simulink model "room"  (R2024b)
settings: Solver=VariableStepAuto  StartTime=0.0  StopTime=172800  RelTol=1e-3
libraries: fl_lib x9, nesl_utility x5, simulink x2
settings Model: Creator=bhalg  LastModifiedBy=bhalg

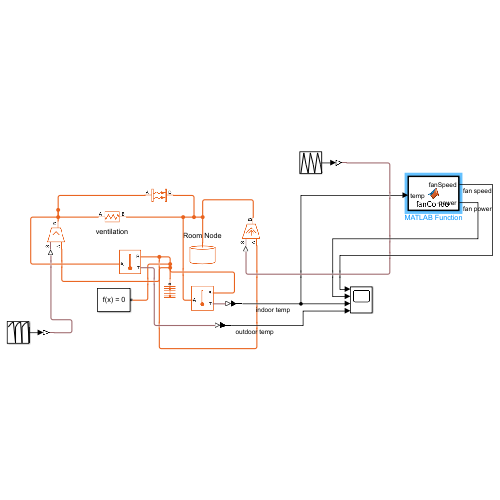
[thumbnail: Simulink's stored preview of the top-level diagram]
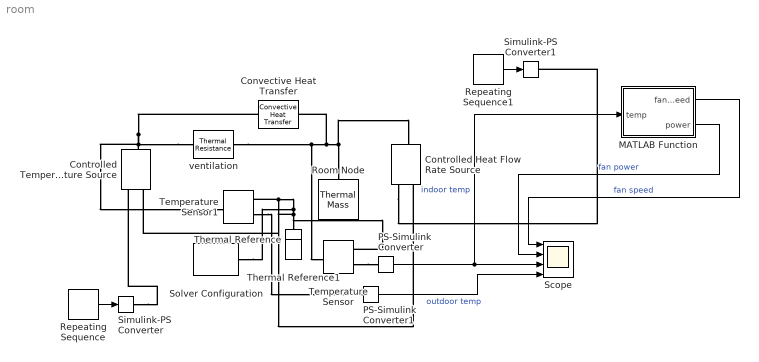
== system room ==
  Controlled Temperature Source : fl_lib/Thermal/Thermal Sources/Controlled Temperature Source
  Controlled Heat Flow Rate Source : fl_lib/Thermal/Thermal Sources/Controlled Heat Flow Rate Source
  Convective Heat Transfer : fl_lib/Thermal/Thermal Elements/Convective Heat Transfer  thermal_type=foundation.enum.constant_variable.constant  area=1 m^2  heat_tr_coeff=2 W/(K*m^2)  min_heat_tr_coeff=1e-3 W/(K*m^2)  T_specify=off  T_priority=None  T=0 K  T_nominal_specify=off  T_nominal_value=1  T_nominal_unit=K  Q_specify=off  Q_priority=None  Q=0 W  Q_nominal_specify=off  Q_nominal_value=1  Q_nominal_unit=W
  MATLAB Function : MATLAB Function  TreatAsAtomicUnit=on
  PS-Simulink Converter : nesl_utility/PS-Simulink Converter  PhysicalDomain=network_engine_domain  SubClassName=ps_output  LeftPortType=input  RightPortType=output  PseudoPeriodic=off  Frequencies=[]  VectorFormat=inherit  Unit=inherit  AffineConversion=off
  PS-Simulink Converter1 : nesl_utility/PS-Simulink Converter  PhysicalDomain=network_engine_domain  SubClassName=ps_output  LeftPortType=input  RightPortType=output  PseudoPeriodic=off  Frequencies=[]  VectorFormat=inherit  Unit=inherit  AffineConversion=off
  Repeating Sequence : simulink/Sources/Repeating Sequence  rep_seq_t=[0 32400 64800 84000]  rep_seq_y=[293 308.15 315.15 227]
  Repeating Sequence1 : simulink/Sources/Repeating Sequence  rep_seq_t=[0 32400 64800 84000]  rep_seq_y=[0 500 200 0]
  Room Node : fl_lib/Thermal/Thermal Elements/Thermal Mass  mass_type=foundation.enum.constant_variable.constant  mass=60 kg  sp_heat=1000 J/(K*kg)  mass_min=1e-6 kg  num_ports=foundation.enum.numPorts2.one  m_specify=off  m_priority=High  m=1 kg  m_nominal_specify=off  m_nominal_value=1  m_nominal_unit=kg  T_specify=on  T_priority=High  T=22 degC  T_nominal_specify=on  T_nominal_value=295.15  T_nominal_unit=K  Q_specify=off  Q_priority=High  Q=0 W  Q_nominal_specify=off  Q_nominal_value=0.1  Q_nominal_unit=W
  Scope : Scope  NumInputPorts=4
  Simulink-PS Converter : nesl_utility/Simulink-PS Converter  PhysicalDomain=network_engine_domain  SubClassName=ps_input  LeftPortType=input  RightPortType=output  PseudoPeriodic=off  Frequencies=[]  NoiseDistribution=none  NoiseParameters=[]  Unit=1  AffineConversion=off  FilteringAndDerivatives=provide  SimscapeFilterOrder=1  InputFilterTimeConstant=0.001  UdotUserProvided=0
  Simulink-PS Converter1 : nesl_utility/Simulink-PS Converter  PhysicalDomain=network_engine_domain  SubClassName=ps_input  LeftPortType=input  RightPortType=output  PseudoPeriodic=off  Frequencies=[]  NoiseDistribution=none  NoiseParameters=[]  Unit=1  AffineConversion=off  FilteringAndDerivatives=provide  SimscapeFilterOrder=1  InputFilterTimeConstant=0.001  UdotUserProvided=0
  Solver Configuration : nesl_utility/Solver Configuration  PhysicalDomain=network_engine_domain  SubClassName=solver  LeftPortType=input  RightPortType=generic  Tones=[]  Harmonics=[]  SimulateNoise=off  Profile=off  UseLocalSampling=off  EnableSwitchedLinearOptims=on  FrequencyDomain=off  UseCCode=off  RelTol=0.001  AbsTol=0.001  MinStep=1e-09  ToWorkspace=off  RevertToSquareIcSolve=off  NumHomotopyIterations=100  PhasorMode=off  PhasorModeNumHarmonics=1  ConsistencySolver=NEWTON_XTOL_AFTER_FTOL  IndexReductionMethod=DerivativeReplacement  DoDC=off  ResidualTolerance=1e-09  ConsistencyTolSource=GLOBAL  ConsistencyAbsTol=0.001  ConsistencyRelTol=0.001  ConsistencyTolFactor=0.001  UseLocalSolver=off  LocalSolverChoice=NE_BACKWARD_EULER_ADVANCER  ResolveIndetEquations=on  FunctionEvalNumThread=1  LocalSolverSampleTime=0.001  DoFixedCost=off  MaxNonlinIter=3  MaxModeIter=2  ComputeImpulses=off  ImpulseIterations=2  LinearAlgebra=auto  LinearAlgebraNumThread=0  EquationFormulation=NE_TIME_EF  DelaysMemoryBudget=1024  AutomaticFiltering=on  FilteringTimeConstant=0.001  PartitionStorageMethod=AS_NEEDED  PartitionMemoryBudget=1024  PartitionMethod=ROBUST  MultibodyUseLocalSolver=off  MultibodyLocalSolverChoice=ODE1  MultibodyLocalSolverSampleTime=0.001
  Temperature Sensor : fl_lib/Thermal/Thermal Sensors/Temperature Sensor  temperature_measure=foundation.enum.MeasurementReference.difference
  Temperature Sensor1 : fl_lib/Thermal/Thermal Sensors/Temperature Sensor  temperature_measure=foundation.enum.MeasurementReference.difference
  Thermal Reference : fl_lib/Thermal/Thermal Elements/Thermal Reference
  Thermal Reference1 : fl_lib/Thermal/Thermal Elements/Thermal Reference
  ventilation : fl_lib/Thermal/Thermal Elements/Thermal Resistance  resistance=2 K/W  T_specify=on  T_priority=High  T=13 degC  T_nominal_specify=on  T_nominal_value=284.15  T_nominal_unit=K  Q_specify=off  Q_priority=High  Q=0 W  Q_nominal_specify=off  Q_nominal_value=0.1  Q_nominal_unit=W
  wires:
  PS-Simulink Converter/1 -> Scope/3, MATLAB Function/1(temp)  "indoor temp"
  PS-Simulink Converter1/1 -> Scope/4  "outdoor temp"
  Repeating Sequence/1 -> Simulink-PS Converter/1
  Repeating Sequence1/1 -> Simulink-PS Converter1/1
  MATLAB Function/2(power) -> Scope/2  "fan power"
  MATLAB Function/1(fanSpeed) -> Scope/1  "fan speed"
  connections:
  ventilation/RConn1 -- Temperature Sensor/LConn1 -- Convective Heat Transfer/RConn1 -- Controlled Heat Flow Rate Source/LConn1 -- Room Node/LConn1
  Temperature Sensor1/RConn1 -- Thermal Reference/LConn1 -- Controlled Temperature Source/RConn2 -- Temperature Sensor/RConn1 -- Solver Configuration/RConn1 -- Controlled Heat Flow Rate Source/RConn2
  Temperature Sensor/RConn2 -- PS-Simulink Converter/LConn1
  ventilation/LConn1 -- Convective Heat Transfer/LConn1 -- Controlled Temperature Source/LConn1 -- Temperature Sensor1/LConn1
  Temperature Sensor1/RConn2 -- PS-Simulink Converter1/LConn1
  Simulink-PS Converter/RConn1 -- Controlled Temperature Source/RConn1
  Controlled Heat Flow Rate Source/RConn1 -- Simulink-PS Converter1/RConn1

== matlab function room/MATLAB Function ==
  data: temp input; fanSpeed output; power output
function [fanSpeed, power] = fanControl(temp)
% fanControl calculates fan speed and power consumption based on temperature
% Inputs:
%   temp - room temperature in °C
% Outputs:
%   fanSpeed - computed fan speed (normalized units)
%   power    - computed power consumption in Watts

% Define parameters
T_ref = 22;       % Reference temperature in °C
S0 = 30;          % Baseline fan speed (normalized units)
k_s = 5;          % Speed gain (units per °C)
P0 = 500;         % Baseline power consumption in Watts
k_p = 20;         % Power gain (W per unit speed increase)

% Calculate fan speed (linear relationship)
fanSpeed = S0 + k_s * (temp - T_ref);

% Calculate power consumption (linear relationship)
power = P0 + k_p * (fanSpeed - S0);
end
